simulink model "SegheriaSCADA2"  (R2024b)
settings: Solver=FixedStepAuto  StartTime=0.0  StopTime=2000  FixedStep=0.025  RelTol=1e-3
values from neighbouring files (symbols this model uses):
  b = t + 2*s    (= 3.6)    [ParametriSegheria.m]    (also in ParametriSegheriaDinamica.m; main_param_CLASSIC.m; main_param_SCADA.m)
  b2 = t2 + 2*s2    (= 10)    [ParametriSegheria.m]    (also in ParametriSegheriaDinamica.m; main_param_CLASSIC.m; main_param_SCADA.m)
  h_index = [70, 80, 90, 100]    [ParametriSegheria.m]    (also in ParametriSegheriaDinamica.m = [80, 90, 100]; main_param_CLASSIC.m = [80, 90, 100, 110]; main_param_SCADA.m = [80, 90, 100, 110])
  h_start_1 = 1    [main_param_CLASSIC.m]
  h_start_2 = 2    [main_param_CLASSIC.m]
  h_start_3 = 3    [main_param_CLASSIC.m]
  h_start_4 = 1    [main_param_CLASSIC.m]
  h_start_5 = 2    [main_param_CLASSIC.m]
  h_start_6 = 3    [main_param_CLASSIC.m]
  i_id = 60    [ParametriSegheria.m]
  i_id2 = 60    [ParametriSegheria.m]
  i_max = 100    [ParametriSegheria.m]
  kc = [0 35 40 50 55 90]    [ParametriSegheria.m]    (also in ParametriSegheriaDinamica.m = [0, 25, 30, 35, 50, 70]; main_param_CLASSIC.m = [0, 25, 30, 35, 50, 70]; main_param_SCADA.m = [0, 25, 30, 35, 50, 70])
  Kt = 2    [ParametriSegheria.m]    (also in ParametriSegheriaDinamica.m = 10000; main_param_CLASSIC.m = 10000; main_param_SCADA.m = 10000)
  Kt2 = 5    [ParametriSegheria.m]    (also in ParametriSegheriaDinamica.m = 4500; main_param_CLASSIC.m = 4500; main_param_SCADA.m = 4500)
  l_index = [20, 30, 40, 50]    [ParametriSegheria.m]    (also in ParametriSegheriaDinamica.m = [30, 40, 50]; main_param_CLASSIC.m = [30, 40, 50, 60]; main_param_SCADA.m = [30, 40, 50, 60])
  l_start_1 = 1    [main_param_CLASSIC.m]
  l_start_2 = 1    [main_param_CLASSIC.m]
  l_start_3 = 1    [main_param_CLASSIC.m]
  l_start_4 = 1    [main_param_CLASSIC.m]
  l_start_5 = 1    [main_param_CLASSIC.m]
  l_start_6 = 1    [main_param_CLASSIC.m]
  Lt = 4    [ParametriSegheria.m]    (also in ParametriSegheriaDinamica.m; main_param_CLASSIC.m; main_param_SCADA.m)
  Mag_D1 = [0 randi([220 500], 1, 40)]    [ParametriSegheria.m]    (also in ParametriSegheriaDinamica.m = [0 randi([200 500], 1, N_log)]; main_param_CLASSIC.m = [0 randi([200 500], 1, N_log)]; main_param_SCADA.m = [0 randi([200 500], 1, N_log)])
  Mag_D2 = [0 randi([220 500], 1, 40)]    [ParametriSegheria.m]    (also in ParametriSegheriaDinamica.m = [0 randi([200 500], 1, N_log)]; main_param_CLASSIC.m = [0 randi([200 500], 1, N_log)]; main_param_SCADA.m = [0 randi([200 500], 1, N_log)])
  Mag_D3 = [0 randi([220 500], 1, 40)]    [ParametriSegheria.m]    (also in ParametriSegheriaDinamica.m = [0 randi([200 500], 1, N_log)]; main_param_CLASSIC.m = [0 randi([200 500], 1, N_log)]; main_param_SCADA.m = [0 randi([200 500], 1, N_log)])
  Mag_legno1 = [0 randi([1 5], 1, 40)]    [ParametriSegheria.m]    (also in ParametriSegheriaDinamica.m = [0 randi([1 5], 1, N_log)]; main_param_CLASSIC.m = [0 randi([1 5], 1, N_log)]; main_param_SCADA.m = [0 randi([1 5], 1, N_log)])
  Mag_legno2 = [0 randi([1 5], 1, 40)]    [ParametriSegheria.m]    (also in ParametriSegheriaDinamica.m = [0 randi([1 5], 1, N_log)]; main_param_CLASSIC.m = [0 randi([1 5], 1, N_log)]; main_param_SCADA.m = [0 randi([1 5], 1, N_log)])
  Mag_legno3 = [0 randi([1 5], 1, 40)]    [ParametriSegheria.m]    (also in ParametriSegheriaDinamica.m = [0 randi([1 5], 1, N_log)]; main_param_CLASSIC.m = [0 randi([1 5], 1, N_log)]; main_param_SCADA.m = [0 randi([1 5], 1, N_log)])
  n_sottili = 4    [ParametriSegheria.m]
  omega = 50    [ParametriSegheria.m]
  omega2 = 3000*(2*pi/60)    (= 314.159265359)    [ParametriSegheria.m]
  SR = Rs/Rm    (= 5.33333333333)    [ParametriSegheria.m]    (also in ParametriSegheriaDinamica.m; main_param_CLASSIC.m; main_param_SCADA.m)
  SR2 = Rc/Rm2    (= 4)    [ParametriSegheria.m]    (also in ParametriSegheriaDinamica.m; main_param_CLASSIC.m; main_param_SCADA.m)
  thrsh = 40    [ParametriSegheria.m]
  Tloss = Tatt+ Tdamp    (= 17.3333333333)    [ParametriSegheria.m]
  Tloss2 = Tatt2+ Tdamp2    (= 66.8318530718)    [ParametriSegheria.m]
libraries: simulink x15, slpidlib x9
(part 1 of 3)
settings Model: Creator=samue  LastModifiedBy=eliasantuari
settings SolverCC: EnableFixedStepZeroCrossing=on

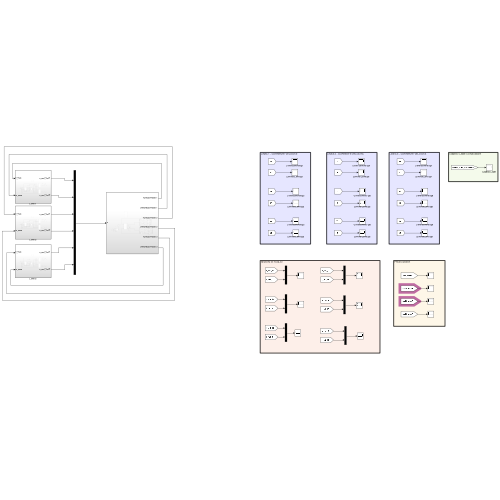
[thumbnail: Simulink's stored preview of the top-level diagram]
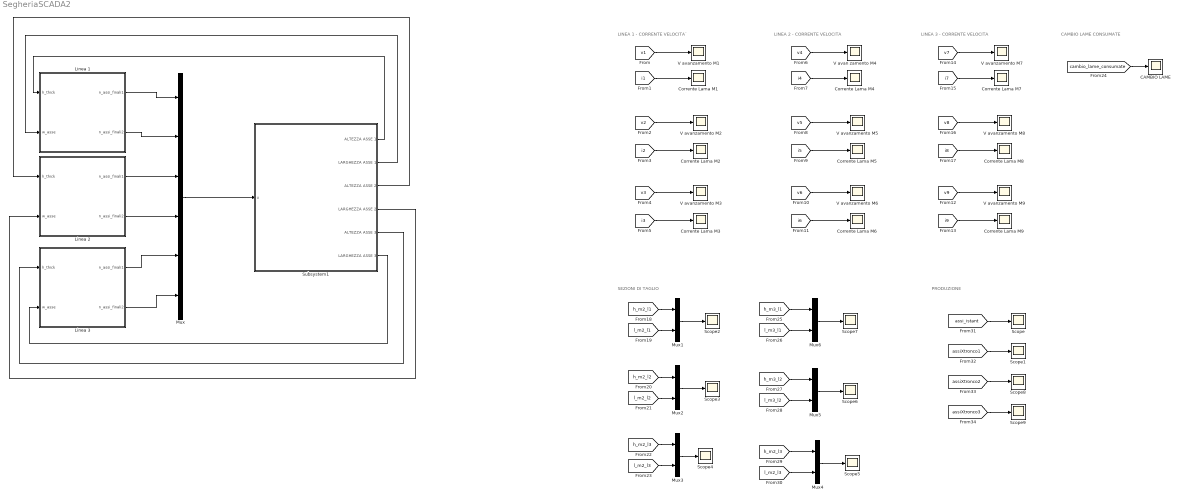
== system SegheriaSCADA2 ==
  note: LINEA 2 - CORRENTE VELOCITA
  note: LINEA 1 - CORRENTE VELOCITA`
  note: LINEA 3 - CORRENTE VELOCITA
  note: SEZIONI DI TAGLIO
  note: CAMBIO LAME CONSUMATE
  note: PRODUZIONE
  CAMBIO LAME : Scope
  Corrente Lama M{1..9} (9 alike) : Scope
  Linea 1 : Subsystem
  Linea 2 : Subsystem
  Linea 3 : Subsystem
  Mux : Mux  Inputs=6
  Mux{1..6} (6 alike) : Mux  Inputs=2
  Scope{,1..9} (10 alike) : Scope
  Subsystem1 : Subsystem
  V avan zamento M4 : Scope
  V avanzamento M{1..3,5..9} (8 alike) : Scope
  wires:
  Linea 2/1(n_assi_finali1) -> Mux/3
  Subsystem1/2(LARGHEZZA ASSE 1) -> Linea 1/2(w_asse)
  Linea 2/2(n_assi_finali2) -> Mux/4
  [i9] -> Corrente Lama M9/1
  [v9] -> V avanzamento M9/1
  [i8] -> Corrente Lama M8/1
  [v7] -> V avanzamento M7/1
  [v8] -> V avanzamento M8/1
  [i7] -> Corrente Lama M7/1
  Subsystem1/6(LARGHEZZA ASSE 3) -> Linea 3/2(w_asse)
  Subsystem1/3(ALTEZZA ASSE 2) -> Linea 2/1(h_thick)
  [i3] -> Corrente Lama M3/1
  [v2] -> V avanzamento M2/1
  [v1] -> V avanzamento M1/1
  Subsystem1/1(ALTEZZA ASSE 1) -> Linea 1/1(h_thick)
  [i2] -> Corrente Lama M2/1
  [i1] -> Corrente Lama M1/1
  Linea 1/1(n_assi_finali1) -> Mux/1
  [v3] -> V avanzamento M3/1
  Mux/1 -> Subsystem1/1(u)
  Linea 3/2(n_assi_finali2) -> Mux/6
  [i5] -> Corrente Lama M5/1
  [v5] -> V avanzamento M5/1
  Linea 3/1(n_assi_finali1) -> Mux/5
  Linea 1/2(n_assi_finali2) -> Mux/2
  [i4] -> Corrente Lama M4/1
  [v4] -> V avan zamento M4/1
  [v6] -> V avanzamento M6/1
  [i6] -> Corrente Lama M6/1
  Subsystem1/5(ALTEZZA ASSE 3) -> Linea 3/1(h_thick)
  Subsystem1/4(LARGHEZZA ASSE 2) -> Linea 2/2(w_asse)
  [cambio_lame_consumate] -> CAMBIO LAME/1
  [l_m2_l1] -> Mux1/2
  [h_m2_l1] -> Mux1/1
  Mux1/1 -> Scope2/1
  [h_m2_l2] -> Mux2/1
  [l_m2_l2] -> Mux2/2
  Mux2/1 -> Scope3/1
  Mux3/1 -> Scope4/1
  [h_m2_l3] -> Mux3/1
  [l_m2_l3] -> Mux3/2
  Mux4/1 -> Scope5/1
  [h_m2_l3] -> Mux4/1
  [l_m2_l3] -> Mux4/2
  Mux5/1 -> Scope6/1
  [h_m3_l2] -> Mux5/1
  [l_m3_l2] -> Mux5/2
  Mux6/1 -> Scope7/1
  [h_m3_l1] -> Mux6/1
  [l_m3_l1] -> Mux6/2
  [assi_istant] -> Scope/1
  [assiXtronco1] -> Scope1/1
  [assiXtronco2] -> Scope8/1
  [assiXtronco3] -> Scope9/1

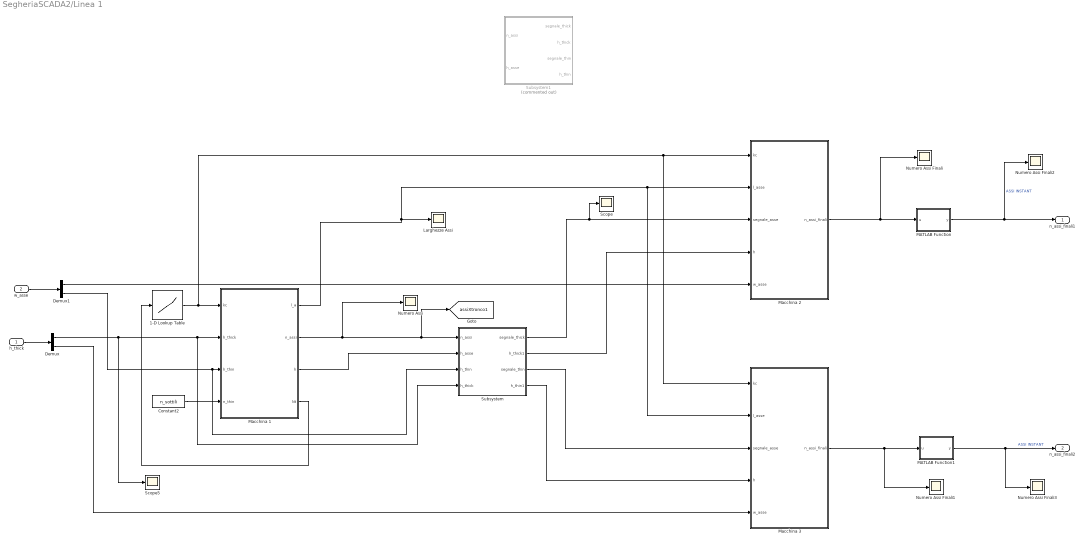
== system SegheriaSCADA2/Linea 1 ==
  h_thick : Inport
  w_asse : Inport  Port=2
  1-D Lookup Table : Lookup_n-D  NumberOfTableDimensions=1  BreakpointsForDimension1=[0 1 2 3 4 5 ]  Table=kc  InternalRulePriority=Speed  RndMeth=Simplest
  Constant2 : Constant  Value=n_sottili
  Demux : Demux  Outputs=2
  Demux1 : Demux  Outputs=2
  Larghezze Assi : Scope
  MATLAB Function : MATLAB Function  TreatAsAtomicUnit=on
  MATLAB Function1 : MATLAB Function  TreatAsAtomicUnit=on
  Macchina 1 : Subsystem
  Macchina 2 : Subsystem
  Macchina 3 : Subsystem
  Numero Assi : Scope
  Numero Assi Finali{,1..3} (4 alike) : Scope
  Scope : Scope
  Scope5 : Scope
  Subsystem : Subsystem
  Subsystem1 : Subsystem  Commented=on
  n_assi_finali1 : Outport
  n_assi_finali2 : Outport  Port=2
  tag scope: assiXtronco1=global
  wires:
  1-D Lookup Table/1 -> Macchina 1/1(kc), Macchina 3/1(kc), Macchina 2/1(kc)
  Macchina 1/1(l_a) -> Macchina 3/2(l_asse), Macchina 2/2(l_asse), Larghezze Assi/1
  Macchina 1/2(n_assi) -> Numero Assi/1, [assiXtronco1], Subsystem/1(n_assi)
  Macchina 1/4(Nt) -> 1-D Lookup Table/1
  Macchina 1/3(h) -> Subsystem/2(h_asse)
  Constant2/1 -> Macchina 1/4(n_thin)
  Macchina 3/1(n_assi_finali) -> Numero Assi Finali1/1, MATLAB Function1/1(u)
  Macchina 2/1(n_assi_finali) -> Numero Assi Finali/1, MATLAB Function/1(u)
  MATLAB Function/1(y) -> Numero Assi Finali2/1, n_assi_finali1/1  "ASSI INSTANT"
  MATLAB Function1/1(y) -> Numero Assi Finali3/1, n_assi_finali2/1  "ASSI INSTANT"
  h_thick/1 -> Demux/1
  Demux/1 -> Scope5/1, Macchina 1/2(h_thick), Subsystem/4(h_thick)
  w_asse/1 -> Demux1/1
  Demux1/1 -> Macchina 2/5(w_asse)
  Demux/2 -> Macchina 3/5(w_asse)
  Demux1/2 -> Macchina 1/3(h_thin), Subsystem/3(h_thin)
  Subsystem/1(segnale_thick) -> Scope/1, Macchina 2/3(segnale_asse)
  Subsystem/2(h_thick1) -> Macchina 2/4(h)
  Subsystem/3(segnale_thin) -> Macchina 3/3(segnale_asse)
  Subsystem/4(h_thin1) -> Macchina 3/4(h)

== system SegheriaSCADA2/Linea 2 ==
  h_thick : Inport
  w_asse : Inport  Port=2
  1-D Lookup Table : Lookup_n-D  NumberOfTableDimensions=1  BreakpointsForDimension1=[0 1 2 3 4 5 ]  Table=kc  InternalRulePriority=Speed  RndMeth=Simplest
  Constant2 : Constant  Value=n_sottili
  Demux : Demux  Outputs=2
  Demux1 : Demux  Outputs=2
  Larghezze Assi : Scope
  MATLAB Function : MATLAB Function  TreatAsAtomicUnit=on
  MATLAB Function1 : MATLAB Function  TreatAsAtomicUnit=on
  Macchina 1 : Subsystem
  Macchina 2 : Subsystem
  Macchina 3 : Subsystem
  Numero Assi : Scope
  Numero Assi Finali{,1..3} (4 alike) : Scope
  Scope5 : Scope
  Subsystem : Subsystem
  Subsystem1 : Subsystem  Commented=on
  n_assi_finali1 : Outport
  n_assi_finali2 : Outport  Port=2
  tag scope: assiXtronco2=global
  wires:
  1-D Lookup Table/1 -> Macchina 1/1(kc), Macchina 3/1(kc), Macchina 2/1(kc)
  Macchina 1/1(l_a) -> Macchina 3/2(l_asse), Macchina 2/2(l_asse), Larghezze Assi/1
  Macchina 1/2(n_assi) -> Numero Assi/1, [assiXtronco2], Subsystem/1(n_assi)
  Macchina 1/4(Nt) -> 1-D Lookup Table/1
  Macchina 1/3(h) -> Subsystem/2(h_asse)
  Constant2/1 -> Macchina 1/4(n_thin)
  Macchina 3/1(n_assi_finali) -> Numero Assi Finali1/1, MATLAB Function1/1(u)
  Macchina 2/1(n_assi_finali) -> Numero Assi Finali/1, MATLAB Function/1(u)
  MATLAB Function/1(y) -> Numero Assi Finali2/1, n_assi_finali1/1  "ASSI INSTANT"
  MATLAB Function1/1(y) -> Numero Assi Finali3/1, n_assi_finali2/1  "ASSI INSTANT"
  h_thick/1 -> Demux/1
  Demux/1 -> Scope5/1, Macchina 1/2(h_thick), Subsystem/4(h_thick)
  w_asse/1 -> Demux1/1
  Demux1/1 -> Macchina 2/5(w_asse)
  Demux/2 -> Macchina 3/5(w_asse)
  Demux1/2 -> Macchina 1/3(h_thin), Subsystem/3(h_thin)
  Subsystem/1(segnale_thick) -> Macchina 2/3(segnale_asse)
  Subsystem/2(h_thick1) -> Macchina 2/4(h)
  Subsystem/3(segnale_thin) -> Macchina 3/3(segnale_asse)
  Subsystem/4(h_thin1) -> Macchina 3/4(h)

== system SegheriaSCADA2/Linea 3 ==
  h_thick : Inport
  w_asse : Inport  Port=2
  1-D Lookup Table : Lookup_n-D  NumberOfTableDimensions=1  BreakpointsForDimension1=[0 1 2 3 4 5 ]  Table=kc  InternalRulePriority=Speed  RndMeth=Simplest
  Constant2 : Constant  Value=n_sottili
  Demux : Demux  Outputs=2
  Demux1 : Demux  Outputs=2
  Larghezze Assi : Scope
  MATLAB Function : MATLAB Function  TreatAsAtomicUnit=on
  MATLAB Function1 : MATLAB Function  TreatAsAtomicUnit=on
  Macchina 1 : Subsystem
  Macchina 2 : Subsystem
  Macchina 3 : Subsystem
  Numero Assi : Scope
  Numero Assi Finali{,1..3} (4 alike) : Scope
  Scope5 : Scope
  Subsystem : Subsystem
  Subsystem1 : Subsystem  Commented=on
  n_assi_finali1 : Outport
  n_assi_finali2 : Outport  Port=2
  tag scope: assiXtronco3=global
  wires:
  Subsystem/4(h_thin1) -> Macchina 3/4(h)
  Subsystem/3(segnale_thin) -> Macchina 3/3(segnale_asse)
  Subsystem/2(h_thick1) -> Macchina 2/4(h)
  Subsystem/1(segnale_thick) -> Macchina 2/3(segnale_asse)
  Demux1/2 -> Subsystem/3(h_thin), Macchina 1/3(h_thin)
  Demux/2 -> Macchina 3/5(w_asse)
  Demux1/1 -> Macchina 2/5(w_asse)
  w_asse/1 -> Demux1/1
  Demux/1 -> Subsystem/4(h_thick), Macchina 1/2(h_thick), Scope5/1
  h_thick/1 -> Demux/1
  MATLAB Function1/1(y) -> n_assi_finali2/1, Numero Assi Finali3/1  "ASSI INSTANT"
  MATLAB Function/1(y) -> n_assi_finali1/1, Numero Assi Finali2/1  "ASSI INSTANT"
  Macchina 2/1(n_assi_finali) -> MATLAB Function/1(u), Numero Assi Finali/1
  Macchina 3/1(n_assi_finali) -> MATLAB Function1/1(u), Numero Assi Finali1/1
  Constant2/1 -> Macchina 1/4(n_thin)
  Macchina 1/3(h) -> Subsystem/2(h_asse)
  Macchina 1/4(Nt) -> 1-D Lookup Table/1
  Macchina 1/2(n_assi) -> [assiXtronco3], Subsystem/1(n_assi), Numero Assi/1
  Macchina 1/1(l_a) -> Larghezze Assi/1, Macchina 2/2(l_asse), Macchina 3/2(l_asse)
  1-D Lookup Table/1 -> Macchina 2/1(kc), Macchina 3/1(kc), Macchina 1/1(kc)

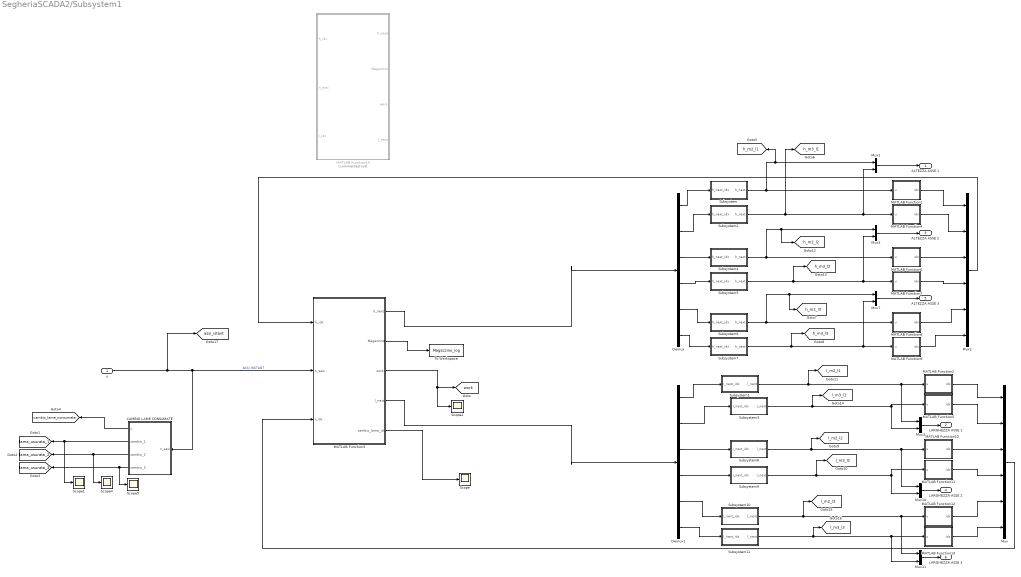
== system SegheriaSCADA2/Subsystem1 ==
  u : Inport
  CAMBIO LAME CONSUMATE : MATLAB Function  TreatAsAtomicUnit=on
  Demux : Demux  Outputs=6
  Demux1 : Demux  Outputs=6
  MATLAB Function1 : MATLAB Function  TreatAsAtomicUnit=on
  MATLAB Function10 : MATLAB Function  TreatAsAtomicUnit=on
  MATLAB Function11 : MATLAB Function  TreatAsAtomicUnit=on
  MATLAB Function12 : MATLAB Function  TreatAsAtomicUnit=on
  MATLAB Function13 : MATLAB Function  TreatAsAtomicUnit=on
  MATLAB Function14 : MATLAB Function  Commented=on  TreatAsAtomicUnit=on
  MATLAB Function2 : MATLAB Function  TreatAsAtomicUnit=on
  MATLAB Function3 : MATLAB Function  TreatAsAtomicUnit=on
  MATLAB Function4 : MATLAB Function  TreatAsAtomicUnit=on
  MATLAB Function5 : MATLAB Function  TreatAsAtomicUnit=on
  MATLAB Function6 : MATLAB Function  TreatAsAtomicUnit=on
  MATLAB Function7 : MATLAB Function  TreatAsAtomicUnit=on
  MATLAB Function8 : MATLAB Function  TreatAsAtomicUnit=on
  MATLAB Function9 : MATLAB Function  TreatAsAtomicUnit=on
  Mux : Mux  Inputs=6
  Mux{1,3,5,7,10..11} (6 alike) : Mux  Inputs=2
  Mux2 : Mux  Inputs=6
  Scope{,1..2,4..5} (5 alike) : Scope
  Subsystem : Subsystem
  Subsystem1 : Subsystem
  Subsystem10 : Subsystem
  Subsystem11 : Subsystem
  Subsystem2 : Subsystem
  Subsystem3 : Subsystem
  Subsystem4 : Subsystem
  Subsystem5 : Subsystem
  Subsystem6 : Subsystem
  Subsystem7 : Subsystem
  Subsystem8 : Subsystem
  Subsystem9 : Subsystem
  To Workspace : ToWorkspace  VariableName=Magazzino_log  SaveFormat=Timeseries  SampleTime=-1
  ALTEZZA ASSE 1 : Outport
  LARGHEZZA ASSE 1 : Outport  Port=2
  ALTEZZA ASSE 2 : Outport  Port=3
  LARGHEZZA ASSE 2 : Outport  Port=4
  ALTEZZA ASSE 3 : Outport  Port=5
  LARGHEZZA ASSE 3 : Outport  Port=6
  tag scope: assi_istant=global, cambio_lame_consumate=global, h_m2_l1=global, h_m2_l2=global, h_m2_l3=global, h_m3_l1=global, h_m3_l2=global, h_m3_l3=global, l_m2_l1=global, l_m2_l2=global, l_m2_l3=global, l_m3_l1=global, l_m3_l2=global, l_m3_l3=global, lama_usurata_1=global, lama_usurata_2=global, lama_usurata_3=global, work=global
  wires:
  Subsystem/1(h_next) -> Mux1/1, [h_m2_l1], MATLAB Function1/1(u)
  Subsystem1/1(l_next) -> [l_m2_l1], Mux3/1, MATLAB Function2/1(u)
  MATLAB Function3/1(h_next) -> Demux/1
  Subsystem2/1(h_next) -> Mux1/2, MATLAB Function4/1(u), [h_m3_l1]
  Demux/2 -> Subsystem2/1(h_next_idx)
  Demux/1 -> Subsystem/1(h_next_idx)
  Mux1/1 -> ALTEZZA ASSE 1/1
  Subsystem3/1(l_next) -> [l_m3_l1], MATLAB Function5/1(u), Mux3/2
  Mux3/1 -> LARGHEZZA ASSE 1/1
  MATLAB Function3/3(work) -> [work], Scope2/1
  Subsystem5/1(h_next) -> [h_m3_l2], Mux5/2, MATLAB Function7/1(u)
  Mux5/1 -> ALTEZZA ASSE 2/1
  Subsystem4/1(h_next) -> [h_m2_l2], Mux5/1, MATLAB Function6/1(u)
  Subsystem7/1(h_next) -> [h_m3_l3], Mux7/2, MATLAB Function9/1(u)
  Mux7/1 -> ALTEZZA ASSE 3/1
  Subsystem6/1(h_next) -> [h_m2_l3], Mux7/1, MATLAB Function8/1(u)
  Demux/3 -> Subsystem4/1(h_next_idx)
  Demux/4 -> Subsystem5/1(h_next_idx)
  Demux/5 -> Subsystem6/1(h_next_idx)
  Demux/6 -> Subsystem7/1(h_next_idx)
  Mux10/1 -> LARGHEZZA ASSE 2/1
  Subsystem9/1(l_next) -> [l_m3_l2], MATLAB Function11/1(u), Mux10/2
  Subsystem8/1(l_next) -> [l_m2_l2], MATLAB Function10/1(u), Mux10/1
  Subsystem10/1(l_next) -> [l_m2_l3], Mux11/1, MATLAB Function12/1(u)
  Subsystem11/1(l_next) -> [l_m3_l3], Mux11/2, MATLAB Function13/1(u)
  Mux11/1 -> LARGHEZZA ASSE 3/1
  MATLAB Function3/4(l_next) -> Demux1/1
  Demux1/1 -> Subsystem1/1(I_next_idx)
  Demux1/2 -> Subsystem3/1(I_next_idx)
  Demux1/3 -> Subsystem8/1(I_next_idx)
  Demux1/4 -> Subsystem9/1(I_next_idx)
  Demux1/5 -> Subsystem10/1(I_next_idx)
  Demux1/6 -> Subsystem11/1(I_next_idx)
  MATLAB Function2/1(idx) -> Mux/1
  MATLAB Function5/1(idx) -> Mux/2
  MATLAB Function10/1(idx) -> Mux/3
  MATLAB Function11/1(idx) -> Mux/4
  MATLAB Function12/1(idx) -> Mux/5
  MATLAB Function13/1(idx) -> Mux/6
  Mux/1 -> MATLAB Function3/3(l_idx)
  MATLAB Function1/1(idx) -> Mux2/1
  MATLAB Function4/1(idx) -> Mux2/2
  MATLAB Function6/1(idx) -> Mux2/3
  MATLAB Function7/1(idx) -> Mux2/4
  MATLAB Function8/1(idx) -> Mux2/5
  MATLAB Function9/1(idx) -> Mux2/6
  Mux2/1 -> MATLAB Function3/1(h_idx)
  u/1 -> [assi_istant], MATLAB Function3/2(n_assi), CAMBIO LAME CONSUMATE/1(n_assi)  "ASSI INSTANT"
  MATLAB Function3/2(Magazzino) -> To Workspace/1
  MATLAB Function3/5(cambio_lama_idx) -> Scope/1
  CAMBIO LAME CONSUMATE/1(y) -> [cambio_lame_consumate]
  CAMBIO LAME CONSUMATE/2(cambio_1) -> Scope1/1, [lama_usurata_1]
  CAMBIO LAME CONSUMATE/4(cambio_3) -> Scope5/1, [lama_usurata_3]
  CAMBIO LAME CONSUMATE/3(cambio_2) -> Scope4/1, [lama_usurata_2]

== system SegheriaSCADA2/Linea 1/Macchina 1 ==
  kc : Inport
  h_thick : Inport  Port=2
  h_thin : Inport  Port=3
  n_thin : Inport  Port=4
  Dinamica Macchina 1 : Subsystem
  Logica Macchina 1 : Subsystem
  l_a : Outport
  n_assi : Outport  Port=2
  h : Outport  Port=3
  Nt : Outport  Port=4
  tag scope: v1=global
  wires:
  kc/1 -> Dinamica Macchina 1/1(kc)
  Dinamica Macchina 1/1(v1) -> [v1], Logica Macchina 1/1(v1)
  Logica Macchina 1/3(Nt) -> Nt/1
  Logica Macchina 1/5(Dt) -> Dinamica Macchina 1/2(Dt)
  Logica Macchina 1/1(n_assi) -> n_assi/1
  Logica Macchina 1/2(l_a) -> l_a/1
  h_thick/1 -> Logica Macchina 1/2(h_thick)
  h_thin/1 -> Logica Macchina 1/3(h_thin)
  n_thin/1 -> Logica Macchina 1/4(n_thin)
  Logica Macchina 1/4(h) -> h/1
  Logica Macchina 1/6(Tronco Finito) -> Dinamica Macchina 1/3(Tronco Finito)

== system SegheriaSCADA2/Linea 1/Macchina 2 ==
  kc : Inport
  l_asse : Inport  Port=2
  segnale_asse : Inport  Port=3
  h : Inport  Port=4
  w_asse : Inport  Port=5
  Ceil : Rounding  Operator=ceil
  Constant2 : Constant  Value=0
  Dinamica Macchina 2 : Subsystem
  Divide : Product  Inputs=*/
  Integrator : Integrator  ExternalReset=falling
  MATLAB Function2 : MATLAB Function  TreatAsAtomicUnit=on
  Memory : Memory
  OR : Logic  Operator=OR  IconShape=distinctive  AllPortsSameDT=off  OutDataTypeStr=boolean
  Scope2 : Scope
  Scope5 : Scope
  Scope8 : Scope
  Switch : Switch  Criteria=u2 > Threshold  SaturateOnIntegerOverflow=off  InputSameDT=off
  w_asse1 : InportShadow  Port=5
  n_assi_finali : Outport
  tag scope: v2=global
  wires:
  Divide/1 -> Ceil/1
  OR/1 -> Switch/2, Memory/1
  Dinamica Macchina 2/1(v1) -> [v2], Integrator/1
  Constant2/1 -> Switch/3
  Switch/1 -> Dinamica Macchina 2/2(kc)
  Integrator/1 -> Scope5/1, MATLAB Function2/1(u)
  MATLAB Function2/2(taglio) -> OR/2, Scope2/1
  h/1 -> Dinamica Macchina 2/3(h)
  l_asse/1 -> MATLAB Function2/3(l_asse), Divide/1
  Ceil/1 -> Scope8/1, Dinamica Macchina 2/1(n_seghe)
  Memory/1 -> Integrator/2
  kc/1 -> Switch/1
  MATLAB Function2/1(y) -> n_assi_finali/1
  w_asse1/1 -> Divide/2
  segnale_asse/1 -> OR/1
  w_asse/1 -> MATLAB Function2/2(w_asse)

== system SegheriaSCADA2/Linea 1/Macchina 3 ==
  kc : Inport
  l_asse : Inport  Port=2
  segnale_asse : Inport  Port=3
  h : Inport  Port=4
  w_asse : Inport  Port=5
  Ceil : Rounding  Operator=ceil
  Constant2 : Constant  Value=0
  Dinamica Macchina 2 : Subsystem
  Divide : Product  Inputs=*/
  Integrator : Integrator  ExternalReset=falling
  MATLAB Function2 : MATLAB Function  TreatAsAtomicUnit=on
  Memory : Memory
  OR : Logic  Operator=OR  IconShape=distinctive  AllPortsSameDT=off  OutDataTypeStr=boolean
  Scope2 : Scope
  Scope5 : Scope
  Scope8 : Scope
  Switch : Switch  Criteria=u2 > Threshold  SaturateOnIntegerOverflow=off  InputSameDT=off
  w_asse1 : InportShadow  Port=5
  n_assi_finali : Outport
  tag scope: v3=global
  wires:
  segnale_asse/1 -> OR/1
  w_asse1/1 -> Divide/2
  MATLAB Function2/1(y) -> n_assi_finali/1
  kc/1 -> Switch/1
  Memory/1 -> Integrator/2
  Ceil/1 -> Dinamica Macchina 2/1(n_seghe), Scope8/1
  l_asse/1 -> Divide/1, MATLAB Function2/3(l_asse)
  h/1 -> Dinamica Macchina 2/3(h)
  MATLAB Function2/2(taglio) -> OR/2, Scope2/1
  Integrator/1 -> MATLAB Function2/1(u), Scope5/1
  Switch/1 -> Dinamica Macchina 2/2(kc)
  Constant2/1 -> Switch/3
  Dinamica Macchina 2/1(v1) -> Integrator/1, [v3]
  OR/1 -> Memory/1, Switch/2
  Divide/1 -> Ceil/1
  w_asse/1 -> MATLAB Function2/2(w_asse)

== system SegheriaSCADA2/Linea 1/Subsystem ==
  n_assi : Inport
  h_asse : Inport  Port=2
  h_thin : Inport  Port=3
  h_thick : Inport  Port=4
  AND : Logic  IconShape=distinctive  AllPortsSameDT=off  OutDataTypeStr=boolean
  Compare To Zero : simulink/Logic and Bit Operations/Compare To Zero  relop=~=  OutDataTypeStr=boolean
  Detect Change : simulink/Logic and Bit Operations/Detect Change  vinit=0  OutDataTypeStr=boolean
  Equal : RelationalOperator  Operator===  OutDataTypeStr=boolean  RndMeth=Simplest  InputSameDT=off
  Equal1 : RelationalOperator  Operator===  OutDataTypeStr=boolean  RndMeth=Simplest  InputSameDT=off
  Scope2 : Scope
  Scope6 : Scope
  Switch{,1..3} (4 alike) : Switch  Criteria=u2 > Threshold  SaturateOnIntegerOverflow=off  InputSameDT=off
  Zero : Constant  Value=0  OutDataTypeStr=Inherit: Inherit via back propagation
  Zero1 : Constant  Value=0  OutDataTypeStr=Inherit: Inherit via back propagation
  segnale_thick : Outport
  h_thick1 : Outport  Port=2
  segnale_thin : Outport  Port=3
  h_thin1 : Outport  Port=4
  wires:
  Detect Change/1 -> Scope2/1, AND/2
  Zero/1 -> Switch/3, Switch1/3
  Switch/1 -> h_thick1/1
  n_assi/1 -> Compare To Zero/1, Detect Change/1
  Compare To Zero/1 -> AND/1
  Switch1/1 -> h_thin1/1
  Zero1/1 -> Switch2/3, Switch3/3
  h_asse/1 -> Equal1/2, Equal/2, Switch/1, Switch1/1
  Switch2/1 -> segnale_thick/1
  AND/1 -> Switch3/1, Switch2/1, Scope6/1
  Switch3/1 -> segnale_thin/1
  h_thick/1 -> Equal/1
  Equal/1 -> Switch/2, Switch2/2
  h_thin/1 -> Equal1/1
  Equal1/1 -> Switch1/2, Switch3/2

== system SegheriaSCADA2/Linea 1/Subsystem1 ==
  n_assi : Inport
  h_asse : Inport  Port=2
  AND : Logic  IconShape=distinctive  AllPortsSameDT=off  OutDataTypeStr=boolean
  Compare To Zero : simulink/Logic and Bit Operations/Compare To Zero  relop=~=  OutDataTypeStr=boolean
  Detect Change : simulink/Logic and Bit Operations/Detect Change  vinit=0  OutDataTypeStr=boolean
  Scope2 : Scope
  Scope6 : Scope
  Switch{,1..3} (4 alike) : Switch  Criteria=u2 > Threshold  Threshold=thrsh  SaturateOnIntegerOverflow=off  InputSameDT=off
  Zero : Constant  Value=0  OutDataTypeStr=Inherit: Inherit via back propagation
  Zero1 : Constant  Value=0  OutDataTypeStr=Inherit: Inherit via back propagation
  h_asse1 : InportShadow  Port=2
  segnale_thick : Outport
  h_thick : Outport  Port=2
  segnale_thin : Outport  Port=3
  h_thin : Outport  Port=4
  wires:
  Detect Change/1 -> Scope2/1, AND/2
  Zero/1 -> Switch1/1, Switch/3
  Switch/1 -> h_thick/1
  n_assi/1 -> Compare To Zero/1, Detect Change/1
  Compare To Zero/1 -> AND/1
  Switch1/1 -> h_thin/1
  Zero1/1 -> Switch2/3, Switch3/1
  h_asse/1 -> Switch/1, Switch/2, Switch1/2, Switch1/3
  Switch2/1 -> segnale_thick/1
  h_asse1/1 -> Switch2/2, Switch3/2
  AND/1 -> Switch3/3, Switch2/1, Scope6/1
  Switch3/1 -> segnale_thin/1

== system SegheriaSCADA2/Linea 2/Macchina 1 ==
  kc : Inport
  h_thick : Inport  Port=2
  h_thin : Inport  Port=3
  n_thin : Inport  Port=4
  Dinamica Macchina 1 : Subsystem
  Logica Macchina 1 : Subsystem
  l_a : Outport
  n_assi : Outport  Port=2
  h : Outport  Port=3
  Nt : Outport  Port=4
  tag scope: v4=global
  wires:
  kc/1 -> Dinamica Macchina 1/1(kc)
  Dinamica Macchina 1/1(v1) -> [v4], Logica Macchina 1/1(v1)
  Logica Macchina 1/3(Nt) -> Nt/1
  Logica Macchina 1/5(Dt) -> Dinamica Macchina 1/2(Dt)
  Logica Macchina 1/1(n_assi) -> n_assi/1
  Logica Macchina 1/2(l_a) -> l_a/1
  h_thick/1 -> Logica Macchina 1/2(h_thick)
  h_thin/1 -> Logica Macchina 1/3(h_thin)
  n_thin/1 -> Logica Macchina 1/4(n_thin)
  Logica Macchina 1/4(h) -> h/1
  Logica Macchina 1/6(Tronco Finito) -> Dinamica Macchina 1/3(Tronco Finito)

== system SegheriaSCADA2/Linea 2/Macchina 2 ==
  kc : Inport
  l_asse : Inport  Port=2
  segnale_asse : Inport  Port=3
  h : Inport  Port=4
  w_asse : Inport  Port=5
  Ceil : Rounding  Operator=ceil
  Constant2 : Constant  Value=0
  Dinamica Macchina 2 : Subsystem
  Divide : Product  Inputs=*/
  Integrator : Integrator  ExternalReset=falling
  MATLAB Function2 : MATLAB Function  TreatAsAtomicUnit=on
  Memory : Memory
  OR : Logic  Operator=OR  IconShape=distinctive  AllPortsSameDT=off  OutDataTypeStr=boolean
  Scope2 : Scope
  Scope5 : Scope
  Scope8 : Scope
  Switch : Switch  Criteria=u2 > Threshold  SaturateOnIntegerOverflow=off  InputSameDT=off
  w_asse1 : InportShadow  Port=5
  n_assi_finali : Outport
  tag scope: v5=global
  wires:
  Divide/1 -> Ceil/1
  OR/1 -> Switch/2, Memory/1
  Dinamica Macchina 2/1(v1) -> [v5], Integrator/1
  Constant2/1 -> Switch/3
  Switch/1 -> Dinamica Macchina 2/2(kc)
  Integrator/1 -> Scope5/1, MATLAB Function2/1(u)
  MATLAB Function2/2(taglio) -> OR/2, Scope2/1
  h/1 -> Dinamica Macchina 2/3(h)
  l_asse/1 -> MATLAB Function2/3(l_asse), Divide/1
  Ceil/1 -> Scope8/1, Dinamica Macchina 2/1(n_seghe)
  Memory/1 -> Integrator/2
  kc/1 -> Switch/1
  MATLAB Function2/1(y) -> n_assi_finali/1
  w_asse1/1 -> Divide/2
  segnale_asse/1 -> OR/1
  w_asse/1 -> MATLAB Function2/2(w_asse)

== system SegheriaSCADA2/Linea 2/Macchina 3 ==
  kc : Inport
  l_asse : Inport  Port=2
  segnale_asse : Inport  Port=3
  h : Inport  Port=4
  w_asse : Inport  Port=5
  Ceil : Rounding  Operator=ceil
  Constant2 : Constant  Value=0
  Dinamica Macchina 2 : Subsystem
  Divide : Product  Inputs=*/
  Integrator : Integrator  ExternalReset=falling
  MATLAB Function2 : MATLAB Function  TreatAsAtomicUnit=on
  Memory : Memory
  OR : Logic  Operator=OR  IconShape=distinctive  AllPortsSameDT=off  OutDataTypeStr=boolean
  Scope2 : Scope
  Scope5 : Scope
  Scope8 : Scope
  Switch : Switch  Criteria=u2 > Threshold  SaturateOnIntegerOverflow=off  InputSameDT=off
  w_asse1 : InportShadow  Port=5
  n_assi_finali : Outport
  tag scope: v6=global
  wires:
  segnale_asse/1 -> OR/1
  w_asse1/1 -> Divide/2
  MATLAB Function2/1(y) -> n_assi_finali/1
  kc/1 -> Switch/1
  Memory/1 -> Integrator/2
  Ceil/1 -> Dinamica Macchina 2/1(n_seghe), Scope8/1
  l_asse/1 -> Divide/1, MATLAB Function2/3(l_asse)
  h/1 -> Dinamica Macchina 2/3(h)
  MATLAB Function2/2(taglio) -> OR/2, Scope2/1
  Integrator/1 -> MATLAB Function2/1(u), Scope5/1
  Switch/1 -> Dinamica Macchina 2/2(kc)
  Constant2/1 -> Switch/3
  Dinamica Macchina 2/1(v1) -> Integrator/1, [v6]
  OR/1 -> Memory/1, Switch/2
  Divide/1 -> Ceil/1
  w_asse/1 -> MATLAB Function2/2(w_asse)

== system SegheriaSCADA2/Linea 2/Subsystem ==
  n_assi : Inport
  h_asse : Inport  Port=2
  h_thin : Inport  Port=3
  h_thick : Inport  Port=4
  AND : Logic  IconShape=distinctive  AllPortsSameDT=off  OutDataTypeStr=boolean
  Compare To Zero : simulink/Logic and Bit Operations/Compare To Zero  relop=~=  OutDataTypeStr=boolean
  Detect Change : simulink/Logic and Bit Operations/Detect Change  vinit=0  OutDataTypeStr=boolean
  Equal : RelationalOperator  Operator===  OutDataTypeStr=boolean  RndMeth=Simplest  InputSameDT=off
  Equal1 : RelationalOperator  Operator===  OutDataTypeStr=boolean  RndMeth=Simplest  InputSameDT=off
  Scope2 : Scope
  Scope6 : Scope
  Switch{,1..3} (4 alike) : Switch  Criteria=u2 > Threshold  SaturateOnIntegerOverflow=off  InputSameDT=off
  Zero : Constant  Value=0  OutDataTypeStr=Inherit: Inherit via back propagation
  Zero1 : Constant  Value=0  OutDataTypeStr=Inherit: Inherit via back propagation
  segnale_thick : Outport
  h_thick1 : Outport  Port=2
  segnale_thin : Outport  Port=3
  h_thin1 : Outport  Port=4
  wires:
  Detect Change/1 -> Scope2/1, AND/2
  Zero/1 -> Switch/3, Switch1/3
  Switch/1 -> h_thick1/1
  n_assi/1 -> Compare To Zero/1, Detect Change/1
  Compare To Zero/1 -> AND/1
  Switch1/1 -> h_thin1/1
  Zero1/1 -> Switch2/3, Switch3/3
  h_asse/1 -> Equal1/2, Equal/2, Switch/1, Switch1/1
  Switch2/1 -> segnale_thick/1
  AND/1 -> Switch3/1, Switch2/1, Scope6/1
  Switch3/1 -> segnale_thin/1
  h_thick/1 -> Equal/1
  Equal/1 -> Switch/2, Switch2/2
  h_thin/1 -> Equal1/1
  Equal1/1 -> Switch1/2, Switch3/2

== system SegheriaSCADA2/Linea 2/Subsystem1 ==
  n_assi : Inport
  h_asse : Inport  Port=2
  AND : Logic  IconShape=distinctive  AllPortsSameDT=off  OutDataTypeStr=boolean
  Compare To Zero : simulink/Logic and Bit Operations/Compare To Zero  relop=~=  OutDataTypeStr=boolean
  Detect Change : simulink/Logic and Bit Operations/Detect Change  vinit=0  OutDataTypeStr=boolean
  Scope2 : Scope
  Scope6 : Scope
  Switch{,1..3} (4 alike) : Switch  Criteria=u2 > Threshold  Threshold=thrsh  SaturateOnIntegerOverflow=off  InputSameDT=off
  Zero : Constant  Value=0  OutDataTypeStr=Inherit: Inherit via back propagation
  Zero1 : Constant  Value=0  OutDataTypeStr=Inherit: Inherit via back propagation
  h_asse1 : InportShadow  Port=2
  segnale_thick : Outport
  h_thick : Outport  Port=2
  segnale_thin : Outport  Port=3
  h_thin : Outport  Port=4
  wires:
  Detect Change/1 -> Scope2/1, AND/2
  Zero/1 -> Switch1/1, Switch/3
  Switch/1 -> h_thick/1
  n_assi/1 -> Compare To Zero/1, Detect Change/1
  Compare To Zero/1 -> AND/1
  Switch1/1 -> h_thin/1
  Zero1/1 -> Switch2/3, Switch3/1
  h_asse/1 -> Switch/1, Switch/2, Switch1/2, Switch1/3
  Switch2/1 -> segnale_thick/1
  h_asse1/1 -> Switch2/2, Switch3/2
  AND/1 -> Switch3/3, Switch2/1, Scope6/1
  Switch3/1 -> segnale_thin/1

== system SegheriaSCADA2/Linea 3/Macchina 1 ==
  kc : Inport
  h_thick : Inport  Port=2
  h_thin : Inport  Port=3
  n_thin : Inport  Port=4
  Dinamica Macchina 1 : Subsystem
  Logica Macchina 1 : Subsystem
  l_a : Outport
  n_assi : Outport  Port=2
  h : Outport  Port=3
  Nt : Outport  Port=4
  tag scope: v7=global
  wires:
  Logica Macchina 1/4(h) -> h/1
  n_thin/1 -> Logica Macchina 1/4(n_thin)
  h_thin/1 -> Logica Macchina 1/3(h_thin)
  h_thick/1 -> Logica Macchina 1/2(h_thick)
  Logica Macchina 1/2(l_a) -> l_a/1
  Logica Macchina 1/1(n_assi) -> n_assi/1
  Logica Macchina 1/5(Dt) -> Dinamica Macchina 1/2(Dt)
  Logica Macchina 1/3(Nt) -> Nt/1
  Dinamica Macchina 1/1(v1) -> Logica Macchina 1/1(v1), [v7]
  kc/1 -> Dinamica Macchina 1/1(kc)
  Logica Macchina 1/6(Tronco Finito) -> Dinamica Macchina 1/3(Tronco Finito)

== system SegheriaSCADA2/Linea 3/Macchina 2 ==
  kc : Inport
  l_asse : Inport  Port=2
  segnale_asse : Inport  Port=3
  h : Inport  Port=4
  w_asse : Inport  Port=5
  Ceil : Rounding  Operator=ceil
  Constant2 : Constant  Value=0
  Dinamica Macchina 2 : Subsystem
  Divide : Product  Inputs=*/
  Integrator : Integrator  ExternalReset=falling
  MATLAB Function2 : MATLAB Function  TreatAsAtomicUnit=on
  Memory : Memory
  OR : Logic  Operator=OR  IconShape=distinctive  AllPortsSameDT=off  OutDataTypeStr=boolean
  Scope2 : Scope
  Scope5 : Scope
  Scope8 : Scope
  Switch : Switch  Criteria=u2 > Threshold  SaturateOnIntegerOverflow=off  InputSameDT=off
  w_asse1 : InportShadow  Port=5
  n_assi_finali : Outport
  tag scope: v8=global
  wires:
  w_asse/1 -> MATLAB Function2/2(w_asse)
  segnale_asse/1 -> OR/1
  w_asse1/1 -> Divide/2
  MATLAB Function2/1(y) -> n_assi_finali/1
  kc/1 -> Switch/1
  Memory/1 -> Integrator/2
  Ceil/1 -> Dinamica Macchina 2/1(n_seghe), Scope8/1
  l_asse/1 -> Divide/1, MATLAB Function2/3(l_asse)
  h/1 -> Dinamica Macchina 2/3(h)
  MATLAB Function2/2(taglio) -> Scope2/1, OR/2
  Integrator/1 -> MATLAB Function2/1(u), Scope5/1
  Switch/1 -> Dinamica Macchina 2/2(kc)
  Constant2/1 -> Switch/3
  Dinamica Macchina 2/1(v1) -> Integrator/1, [v8]
  OR/1 -> Memory/1, Switch/2
  Divide/1 -> Ceil/1

== system SegheriaSCADA2/Linea 3/Macchina 3 ==
  kc : Inport
  l_asse : Inport  Port=2
  segnale_asse : Inport  Port=3
  h : Inport  Port=4
  w_asse : Inport  Port=5
  Ceil : Rounding  Operator=ceil
  Constant2 : Constant  Value=0
  Dinamica Macchina 2 : Subsystem
  Divide : Product  Inputs=*/
  Integrator : Integrator  ExternalReset=falling
  MATLAB Function2 : MATLAB Function  TreatAsAtomicUnit=on
  Memory : Memory
  OR : Logic  Operator=OR  IconShape=distinctive  AllPortsSameDT=off  OutDataTypeStr=boolean
  Scope2 : Scope
  Scope5 : Scope
  Scope8 : Scope
  Switch : Switch  Criteria=u2 > Threshold  SaturateOnIntegerOverflow=off  InputSameDT=off
  w_asse1 : InportShadow  Port=5
  n_assi_finali : Outport
  tag scope: v9=global
  wires:
  w_asse/1 -> MATLAB Function2/2(w_asse)
  Divide/1 -> Ceil/1
  OR/1 -> Switch/2, Memory/1
  Dinamica Macchina 2/1(v1) -> [v9], Integrator/1
  Constant2/1 -> Switch/3
  Switch/1 -> Dinamica Macchina 2/2(kc)
  Integrator/1 -> Scope5/1, MATLAB Function2/1(u)
  MATLAB Function2/2(taglio) -> Scope2/1, OR/2
  h/1 -> Dinamica Macchina 2/3(h)
  l_asse/1 -> MATLAB Function2/3(l_asse), Divide/1
  Ceil/1 -> Scope8/1, Dinamica Macchina 2/1(n_seghe)
  Memory/1 -> Integrator/2
  kc/1 -> Switch/1
  MATLAB Function2/1(y) -> n_assi_finali/1
  w_asse1/1 -> Divide/2
  segnale_asse/1 -> OR/1

== system SegheriaSCADA2/Linea 3/Subsystem ==
  n_assi : Inport
  h_asse : Inport  Port=2
  h_thin : Inport  Port=3
  h_thick : Inport  Port=4
  AND : Logic  IconShape=distinctive  AllPortsSameDT=off  OutDataTypeStr=boolean
  Compare To Zero : simulink/Logic and Bit Operations/Compare To Zero  relop=~=  OutDataTypeStr=boolean
  Detect Change : simulink/Logic and Bit Operations/Detect Change  vinit=0  OutDataTypeStr=boolean
  Equal : RelationalOperator  Operator===  OutDataTypeStr=boolean  RndMeth=Simplest  InputSameDT=off
  Equal1 : RelationalOperator  Operator===  OutDataTypeStr=boolean  RndMeth=Simplest  InputSameDT=off
  Scope2 : Scope
  Scope6 : Scope
  Switch{,1..3} (4 alike) : Switch  Criteria=u2 > Threshold  SaturateOnIntegerOverflow=off  InputSameDT=off
  Zero : Constant  Value=0  OutDataTypeStr=Inherit: Inherit via back propagation
  Zero1 : Constant  Value=0  OutDataTypeStr=Inherit: Inherit via back propagation
  segnale_thick : Outport
  h_thick1 : Outport  Port=2
  segnale_thin : Outport  Port=3
  h_thin1 : Outport  Port=4
  wires:
  Equal1/1 -> Switch3/2, Switch1/2
  h_thin/1 -> Equal1/1
  Equal/1 -> Switch2/2, Switch/2
  h_thick/1 -> Equal/1
  Switch3/1 -> segnale_thin/1
  AND/1 -> Scope6/1, Switch2/1, Switch3/1
  Switch2/1 -> segnale_thick/1
  h_asse/1 -> Switch1/1, Switch/1, Equal/2, Equal1/2
  Zero1/1 -> Switch3/3, Switch2/3
  Switch1/1 -> h_thin1/1
  Compare To Zero/1 -> AND/1
  n_assi/1 -> Detect Change/1, Compare To Zero/1
  Switch/1 -> h_thick1/1
  Zero/1 -> Switch1/3, Switch/3
  Detect Change/1 -> AND/2, Scope2/1

== system SegheriaSCADA2/Linea 3/Subsystem1 ==
  n_assi : Inport
  h_asse : Inport  Port=2
  AND : Logic  IconShape=distinctive  AllPortsSameDT=off  OutDataTypeStr=boolean
  Compare To Zero : simulink/Logic and Bit Operations/Compare To Zero  relop=~=  OutDataTypeStr=boolean
  Detect Change : simulink/Logic and Bit Operations/Detect Change  vinit=0  OutDataTypeStr=boolean
  Scope2 : Scope
  Scope6 : Scope
  Switch{,1..3} (4 alike) : Switch  Criteria=u2 > Threshold  Threshold=thrsh  SaturateOnIntegerOverflow=off  InputSameDT=off
  Zero : Constant  Value=0  OutDataTypeStr=Inherit: Inherit via back propagation
  Zero1 : Constant  Value=0  OutDataTypeStr=Inherit: Inherit via back propagation
  h_asse1 : InportShadow  Port=2
  segnale_thick : Outport
  h_thick : Outport  Port=2
  segnale_thin : Outport  Port=3
  h_thin : Outport  Port=4
  wires:
  Switch3/1 -> segnale_thin/1
  AND/1 -> Scope6/1, Switch2/1, Switch3/3
  h_asse1/1 -> Switch3/2, Switch2/2
  Switch2/1 -> segnale_thick/1
  h_asse/1 -> Switch1/3, Switch1/2, Switch/2, Switch/1
  Zero1/1 -> Switch3/1, Switch2/3
  Switch1/1 -> h_thin/1
  Compare To Zero/1 -> AND/1
  n_assi/1 -> Detect Change/1, Compare To Zero/1
  Switch/1 -> h_thick/1
  Zero/1 -> Switch/3, Switch1/1
  Detect Change/1 -> AND/2, Scope2/1

== system SegheriaSCADA2/Subsystem1/Subsystem ==
  h_next_idx : Inport
  Constant4 : Constant  Value=h_index
  Constant7 : Constant  Value=h_start_1
  Memory : Memory
  SELEZIONE ALTEZZA : Selector  InputPortWidth=length(h_index)  IndexOptions=Index vector (port)  Indices=[1 3]  OutputSizes=1
  Switch1 : Switch  Criteria=u2 > Threshold  SaturateOnIntegerOverflow=off  InputSameDT=off
  h_next : Outport
  wires:
  h_next_idx/1 -> Memory/1
  Constant7/1 -> Switch1/3
  Memory/1 -> Switch1/2, Switch1/1
  SELEZIONE ALTEZZA/1 -> h_next/1
  Constant4/1 -> SELEZIONE ALTEZZA/1
  Switch1/1 -> SELEZIONE ALTEZZA/2

== system SegheriaSCADA2/Subsystem1/Subsystem1 ==
  I_next_idx : Inport
  Constant5 : Constant  Value=l_index
  Constant8 : Constant  Value=l_start_1
  Memory1 : Memory
  SELEZIONE LUNGHEZZA : Selector  InputPortWidth=length(h_index)  IndexOptions=Index vector (port)  Indices=[1 3]  OutputSizes=1
  Switch2 : Switch  Criteria=u2 > Threshold  SaturateOnIntegerOverflow=off  InputSameDT=off
  l_next : Outport
  wires:
  Memory1/1 -> Switch2/1, Switch2/2
  SELEZIONE LUNGHEZZA/1 -> l_next/1
  Switch2/1 -> SELEZIONE LUNGHEZZA/2
  Constant5/1 -> SELEZIONE LUNGHEZZA/1
  I_next_idx/1 -> Memory1/1
  Constant8/1 -> Switch2/3

== system SegheriaSCADA2/Subsystem1/Subsystem10 ==
  I_next_idx : Inport
  Constant5 : Constant  Value=l_index
  Constant8 : Constant  Value=l_start_3
  Memory1 : Memory
  SELEZIONE LUNGHEZZA : Selector  InputPortWidth=length(h_index)  IndexOptions=Index vector (port)  Indices=[1 3]  OutputSizes=1
  Switch2 : Switch  Criteria=u2 > Threshold  SaturateOnIntegerOverflow=off  InputSameDT=off
  l_next : Outport
  wires:
  Memory1/1 -> Switch2/1, Switch2/2
  SELEZIONE LUNGHEZZA/1 -> l_next/1
  Switch2/1 -> SELEZIONE LUNGHEZZA/2
  Constant5/1 -> SELEZIONE LUNGHEZZA/1
  I_next_idx/1 -> Memory1/1
  Constant8/1 -> Switch2/3

== system SegheriaSCADA2/Subsystem1/Subsystem11 ==
  I_next_idx : Inport
  Constant5 : Constant  Value=l_index
  Constant8 : Constant  Value=l_start_6
  Memory1 : Memory
  SELEZIONE LUNGHEZZA : Selector  InputPortWidth=length(h_index)  IndexOptions=Index vector (port)  Indices=[1 3]  OutputSizes=1
  Switch2 : Switch  Criteria=u2 > Threshold  SaturateOnIntegerOverflow=off  InputSameDT=off
  l_next : Outport
  wires:
  Constant8/1 -> Switch2/3
  I_next_idx/1 -> Memory1/1
  Constant5/1 -> SELEZIONE LUNGHEZZA/1
  Switch2/1 -> SELEZIONE LUNGHEZZA/2
  SELEZIONE LUNGHEZZA/1 -> l_next/1
  Memory1/1 -> Switch2/2, Switch2/1

== system SegheriaSCADA2/Subsystem1/Subsystem2 ==
  h_next_idx : Inport
  Constant4 : Constant  Value=h_index
  Constant7 : Constant  Value=h_start_4
  Memory : Memory
  SELEZIONE ALTEZZA : Selector  InputPortWidth=length(h_index)  IndexOptions=Index vector (port)  Indices=[1 3]  OutputSizes=1
  Switch1 : Switch  Criteria=u2 > Threshold  SaturateOnIntegerOverflow=off  InputSameDT=off
  h_next : Outport
  wires:
  Switch1/1 -> SELEZIONE ALTEZZA/2
  Constant4/1 -> SELEZIONE ALTEZZA/1
  SELEZIONE ALTEZZA/1 -> h_next/1
  Memory/1 -> Switch1/1, Switch1/2
  Constant7/1 -> Switch1/3
  h_next_idx/1 -> Memory/1

== system SegheriaSCADA2/Subsystem1/Subsystem3 ==
  I_next_idx : Inport
  Constant1 : Constant  Value=l_start_4
  Constant5 : Constant  Value=l_index
  Memory1 : Memory
  SELEZIONE LUNGHEZZA : Selector  InputPortWidth=length(h_index)  IndexOptions=Index vector (port)  Indices=[1 3]  OutputSizes=1
  Switch2 : Switch  Criteria=u2 > Threshold  SaturateOnIntegerOverflow=off  InputSameDT=off
  l_next : Outport
  wires:
  Constant1/1 -> Switch2/3
  I_next_idx/1 -> Memory1/1
  Constant5/1 -> SELEZIONE LUNGHEZZA/1
  Switch2/1 -> SELEZIONE LUNGHEZZA/2
  SELEZIONE LUNGHEZZA/1 -> l_next/1
  Memory1/1 -> Switch2/2, Switch2/1

== system SegheriaSCADA2/Subsystem1/Subsystem4 ==
  h_next_idx : Inport
  Constant4 : Constant  Value=h_index
  Constant7 : Constant  Value=h_start_2
  Memory : Memory
  SELEZIONE ALTEZZA : Selector  InputPortWidth=length(h_index)  IndexOptions=Index vector (port)  Indices=[1 3]  OutputSizes=1
  Switch1 : Switch  Criteria=u2 > Threshold  SaturateOnIntegerOverflow=off  InputSameDT=off
  h_next : Outport
  wires:
  h_next_idx/1 -> Memory/1
  Constant7/1 -> Switch1/3
  Memory/1 -> Switch1/2, Switch1/1
  SELEZIONE ALTEZZA/1 -> h_next/1
  Constant4/1 -> SELEZIONE ALTEZZA/1
  Switch1/1 -> SELEZIONE ALTEZZA/2

== system SegheriaSCADA2/Subsystem1/Subsystem5 ==
  h_next_idx : Inport
  Constant4 : Constant  Value=h_index
  Constant7 : Constant  Value=h_start_5
  Memory : Memory
  SELEZIONE ALTEZZA : Selector  InputPortWidth=length(h_index)  IndexOptions=Index vector (port)  Indices=[1 3]  OutputSizes=1
  Switch1 : Switch  Criteria=u2 > Threshold  SaturateOnIntegerOverflow=off  InputSameDT=off
  h_next : Outport
  wires:
  Switch1/1 -> SELEZIONE ALTEZZA/2
  Constant4/1 -> SELEZIONE ALTEZZA/1
  SELEZIONE ALTEZZA/1 -> h_next/1
  Memory/1 -> Switch1/1, Switch1/2
  Constant7/1 -> Switch1/3
  h_next_idx/1 -> Memory/1

== system SegheriaSCADA2/Subsystem1/Subsystem6 ==
  h_next_idx : Inport
  Constant4 : Constant  Value=h_index
  Constant7 : Constant  Value=h_start_3
  Memory : Memory
  SELEZIONE ALTEZZA : Selector  InputPortWidth=length(h_index)  IndexOptions=Index vector (port)  Indices=[1 3]  OutputSizes=1
  Switch1 : Switch  Criteria=u2 > Threshold  SaturateOnIntegerOverflow=off  InputSameDT=off
  h_next : Outport
  wires:
  h_next_idx/1 -> Memory/1
  Constant7/1 -> Switch1/3
  Memory/1 -> Switch1/2, Switch1/1
  SELEZIONE ALTEZZA/1 -> h_next/1
  Constant4/1 -> SELEZIONE ALTEZZA/1
  Switch1/1 -> SELEZIONE ALTEZZA/2

== system SegheriaSCADA2/Subsystem1/Subsystem7 ==
  h_next_idx : Inport
  Constant4 : Constant  Value=h_index
  Constant7 : Constant  Value=h_start_6
  Memory : Memory
  SELEZIONE ALTEZZA : Selector  InputPortWidth=length(h_index)  IndexOptions=Index vector (port)  Indices=[1 3]  OutputSizes=1
  Switch1 : Switch  Criteria=u2 > Threshold  SaturateOnIntegerOverflow=off  InputSameDT=off
  h_next : Outport
  wires:
  Switch1/1 -> SELEZIONE ALTEZZA/2
  Constant4/1 -> SELEZIONE ALTEZZA/1
  SELEZIONE ALTEZZA/1 -> h_next/1
  Memory/1 -> Switch1/1, Switch1/2
  Constant7/1 -> Switch1/3
  h_next_idx/1 -> Memory/1

== system SegheriaSCADA2/Subsystem1/Subsystem8 ==
  I_next_idx : Inport
  Constant5 : Constant  Value=l_index
  Constant8 : Constant  Value=l_start_2
  Memory1 : Memory
  SELEZIONE LUNGHEZZA : Selector  InputPortWidth=length(h_index)  IndexOptions=Index vector (port)  Indices=[1 3]  OutputSizes=1
  Switch2 : Switch  Criteria=u2 > Threshold  SaturateOnIntegerOverflow=off  InputSameDT=off
  l_next : Outport
  wires:
  Constant8/1 -> Switch2/3
  I_next_idx/1 -> Memory1/1
  Constant5/1 -> SELEZIONE LUNGHEZZA/1
  Switch2/1 -> SELEZIONE LUNGHEZZA/2
  SELEZIONE LUNGHEZZA/1 -> l_next/1
  Memory1/1 -> Switch2/2, Switch2/1

== system SegheriaSCADA2/Subsystem1/Subsystem9 ==
  I_next_idx : Inport
  Constant5 : Constant  Value=l_index
  Constant8 : Constant  Value=l_start_5
  Memory1 : Memory
  SELEZIONE LUNGHEZZA : Selector  InputPortWidth=length(h_index)  IndexOptions=Index vector (port)  Indices=[1 3]  OutputSizes=1
  Switch2 : Switch  Criteria=u2 > Threshold  SaturateOnIntegerOverflow=off  InputSameDT=off
  l_next : Outport
  wires:
  Memory1/1 -> Switch2/1, Switch2/2
  SELEZIONE LUNGHEZZA/1 -> l_next/1
  Switch2/1 -> SELEZIONE LUNGHEZZA/2
  Constant5/1 -> SELEZIONE LUNGHEZZA/1
  I_next_idx/1 -> Memory1/1
  Constant8/1 -> Switch2/3

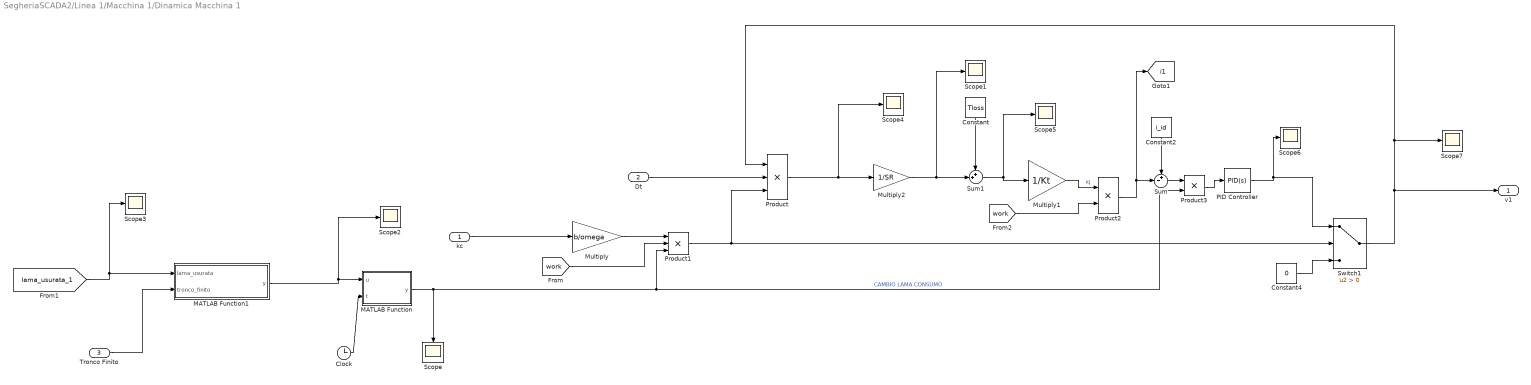
== system SegheriaSCADA2/Linea 1/Macchina 1/Dinamica Macchina 1 ==
  kc : Inport
  Dt : Inport  Port=2
  Tronco Finito : Inport  Port=3
  Clock : Clock
  Constant : Constant  Value=Tloss
  Constant2 : Constant  Value=i_id
  Constant4 : Constant  Value=0
  MATLAB Function : MATLAB Function  TreatAsAtomicUnit=on
  MATLAB Function1 : MATLAB Function  TreatAsAtomicUnit=on
  Multiply : Gain  Gain=b/omega
  Multiply1 : Gain  Gain=1/Kt
  Multiply2 : Gain  Gain=1/SR
  PID Controller : slpidlib/PID Controller  Controller=PID  Form=Parallel  TimeDomain=Continuous-time  UseExternalTs=off  SampleTime=-1  IntegratorMethod=Forward Euler  FilterMethod=Forward Euler  ControllerParametersSource=internal  P=0  I=0.0048685791703887  UseKiTs=off  D=0  UseExternalDerivativeSource=off  N=100  UseFilter=on  TunerSelectOption=Transfer Function Based (PID Tuner App)  InitialConditionSource=internal  InitialConditionForIntegrator=0  InitialConditionForFilter=0  DifferentiatorICPrevScaledInput=0  ExternalReset=none  TrackingMode=off  Kt=1  LimitOutput=on  SatLimitsSource=internal  UpperSaturationLimit=i_max  LowerSaturationLimit=-inf  LinearizeAsGain=on  AntiWindupMode=none  Kb=1  LimitIntegrator=off  UpperIntegratorSaturationLimit=inf  LowerIntegratorSaturationLimit=-inf  POutMin=[]  POutMax=[]  IOutMin=[]  IOutMax=[]  DOutMin=[]  DOutMax=[]  NOutMin=[]  NOutMax=[]  SumOutMin=[]  SumOutMax=[]  SaturationOutMin=[]  SaturationOutMax=[]  PParamMin=[]  PParamMax=[]  IParamMin=[]  IParamMax=[]  DParamMin=[]  DParamMax=[]  NParamMin=[]  NParamMax=[]  KbParamMin=[]  KbParamMax=[]  KtParamMin=[]  KtParamMax=[]  KbOutMin=[]  KbOutMax=[]  KtOutMin=[]  KtOutMax=[]  IntegratorOutMin=[]  IntegratorOutMax=[]  FilterOutMin=[]  FilterOutMax=[]  SumI1OutMin=[]  SumI1OutMax=[]  SumI2OutMin=[]  SumI2OutMax=[]  SumI3OutMin=[]  SumI3OutMax=[]  SumI4OutMin=[]  SumI4OutMax=[]  SumDOutMin=[]  SumDOutMax=[]  DifferentiatorOutMin=[]  DifferentiatorOutMax=[]  FilterDiffOutCoefMin=[]  FilterDiffOutCoefMax=[]  ReciprocalOutMin=[]  ReciprocalOutMax=[]  SumDenOutMin=[]  SumDenOutMax=[]  SumNumOutMin=[]  SumNumOutMax=[]  DivideOutMin=[]  DivideOutMax=[]  UdiffTsProdOutMin=[]  UdiffTsProdOutMax=[]  NTsProdOutMin=[]  NTsProdOutMax=[]  UintegralTsProdOutMin=[]  UintegralTsProdOutMax=[]  UngainTsProdOutMin=[]  UngainTsProdOutMax=[]  ClampingZeroOutDataTypeStr=Inherit: Inherit via back propagation  ClampingZeroOutMin=[]  ClampingZeroOutMax=[]  FilterDenConstantOutDataTypeStr=Inherit: Inherit via back propagation  FilterDenConstantOutMin=[]  FilterDenConstantOutMax=[]  PCopyOutDataTypeStr=Inherit: Inherit via back propagation  PCopyOutMin=[]  PCopyOutMax=[]  NCopyOutDataTypeStr=Inherit: Inherit via back propagation  NCopyOutMin=[]  NCopyOutMax=[]  IntegratorContinuousStateAttributes=''  IntegratorStateMustResolveToSignalObject=off  IntegratorRTWStateStorageClass=Auto  FilterContinuousStateAttributes=''  FilterStateMustResolveToSignalObject=off  FilterRTWStateStorageClass=Auto  ParallelPVariant=InternalParameters  IdealPVariant=Disabled  IVariant=InternalParameters  DVariant=InternalParameters  IntegratorVariant=Continuous  SatVariant=Enabled  AWVariant=Passthrough  PCopyVariant=Disabled  TRVariant=Disabled  FdbkBlocksVariant=Forward  IdealPFdbkVariant=Disabled  SatFdbkVariant=Disabled  DerivativeFilterVariant=ContFilter  NVariant=InternalParameters  NCopyVariant=Disabled  FilterICVariant=InternalICsFilter  IntegratorICVariant=InternalICs  ExternalResetVariant=Disabled  TRSumVariant=Passthrough  SumFdbkVariant=Disabled  SumVariant=Sum_PID  TsampFilterVariant=InternalTs  TsampNgainVariant=Passthrough  TsampIntegralVariant=Disabled_SignalSpec  ExternalSaturationOutDataTypeStr=Inherit: Same as second input  DerivativeSourceVariant=ErrorSignal  PreIntVariant=InternalPreInt
  Product : Product  Inputs=3
  Product1 : Product  Inputs=3
  Product2 : Product
  Product3 : Product
  Scope{,1..7} (8 alike) : Scope
  Sum : Sum  Inputs=+-|
  Sum1 : Sum  Inputs=++|
  Switch1 : Switch  Criteria=u2 > Threshold  SaturateOnIntegerOverflow=off  InputSameDT=off
  v1 : Outport
  tag scope: i1=global
  wires:
  Constant4/1 -> Switch1/3
  Product/1 -> Scope4/1, Multiply2/1
  Multiply1/1 -> Product2/1  "iq"
  kc/1 -> Multiply/1
  Switch1/1 -> v1/1, Scope7/1, Product/1
  Multiply2/1 -> Sum1/2, Scope1/1
  Sum1/1 -> Scope5/1, Multiply1/1
  Constant/1 -> Sum1/1
  Dt/1 -> Product/2
  Multiply/1 -> Product1/1
  Product1/1 -> Switch1/2, Product/3
  [work] -> Product1/2
  Clock/1 -> MATLAB Function/2(t)
  MATLAB Function/1(y) -> Product3/2, Product1/3, Scope/1  "CAMBIO LAMA CONSUMO"
  [lama_usurata_1] -> MATLAB Function1/1(lama_usurata), Scope3/1
  MATLAB Function1/1(y) -> Scope2/1, MATLAB Function/1(u)
  Tronco Finito/1 -> MATLAB Function1/2(tronco_finito)
  Product2/1 -> [i1], Sum/2
  [work] -> Product2/2
  PID Controller/1 -> Scope6/1, Switch1/1
  Constant2/1 -> Sum/1
  Sum/1 -> Product3/1
  Product3/1 -> PID Controller/1
